simulink model "cooler_simple_model_fmu"  (R2022b)
settings: Solver=FixedStepAuto  StartTime=0.0  StopTime=10.0  FixedStep=0.01  RelTol=1e-3
settings Model: Creator=Kumar  LastModifiedBy=Kumar
settings ModelReferenceCC: EnableRefExpFcnMdlSchedulingChecks=on

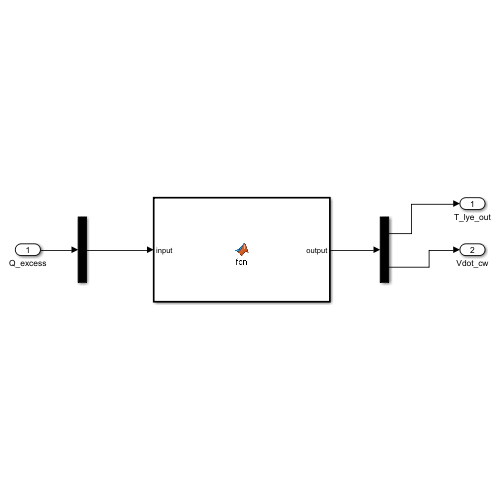
[thumbnail: Simulink's stored preview of the top-level diagram]
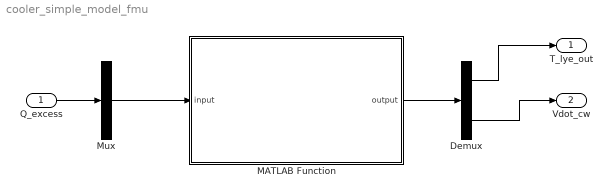
== system cooler_simple_model_fmu ==
  Q_excess : Inport
  Demux : Demux  Outputs=2
  MATLAB Function : MATLAB Function  TreatAsAtomicUnit=on
  Mux : Mux  Inputs=1
  T_lye_out : Outport
  Vdot_cw : Outport  Port=2
  wires:
  MATLAB Function/1(output) -> Demux/1
  Mux/1 -> MATLAB Function/1(input)
  Demux/1 -> T_lye_out/1
  Demux/2 -> Vdot_cw/1
  Q_excess/1 -> Mux/1

== matlab function cooler_simple_model_fmu/MATLAB Function ==
  data: output output; input input
function output = fcn(input)

%% Parameter
T_cw_in     = 293.15;     % K
T_cw_out    = 298.15; % Initial condition
T_el        = 353.15; % Temperature of the electrolyzer
Cp_lye      = 4.2;     % KJ/KgK
Cp_cw       = 4.2;     % KJ/KgK
rho_cw      = 1000;     % kg/m³
rho_lye     = 1230;     % kg/m³
%% Steuergrößen auslesen
%T_lye_in    = input(1);   % Temp in K
Q_dot    = input(1);    % Vol flow in lph

  

%% Modellgleichungen
% Hilfsgleichungen

%Q_dot = (rho_lye * Vdot_lye * Cp_lye * (T_lye_in - T_el)) ;
Vdot_cw = abs(Q_dot/(rho_cw * Cp_cw *(T_cw_in - T_cw_out)));
T_lye_out = T_el;
%Vdot_lye_out = Vdot_lye;
%% Ausgänge
output = [T_lye_out,Vdot_cw];
